simulink model "PID_DC_MOTOR_methods"  (R2016a)
settings: Solver=VariableStepAuto  StartTime=0.0  StopTime=10.0  RelTol=1e-3
InitFcn:
  | J = 0.02;
  | b = 0.05;
  | Ke = 0.1;
  | Kt = 0.2;
  | R = 3;
  | L = 0.5;
  | 
  | thetha_dot0 = 0;
  | i0 = 0;
  | 
libraries: simulink x3
settings Model: Creator=hp  LastModifiedBy=hp

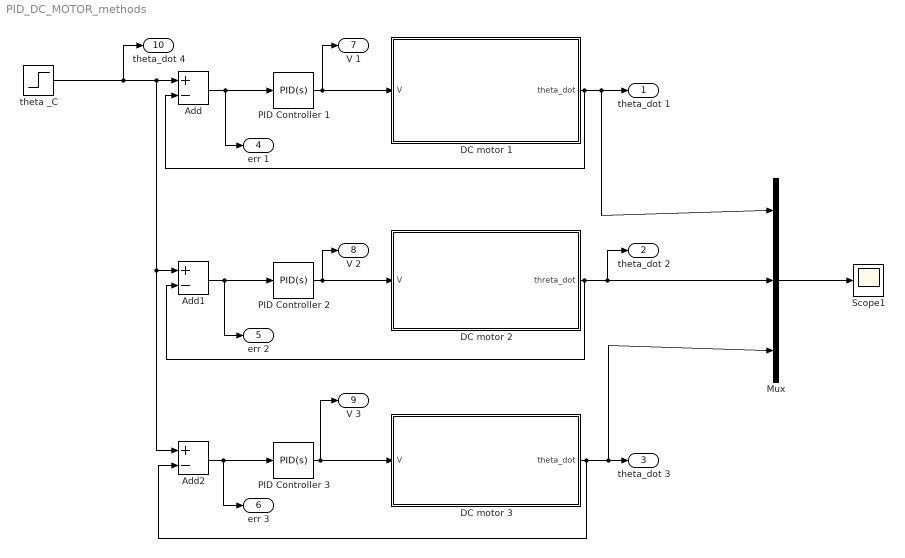
== system PID_DC_MOTOR_methods ==
  Add : Sum  Inputs=+-
  Add1 : Sum  Inputs=+-
  Add2 : Sum  Inputs=+-
  DC motor 1 : Subsystem
  DC motor 2 : Subsystem
  "DC motor 3 " : Subsystem
  Mux : Mux  Inputs=3
  PID Controller 1 : simulink/Continuous/PID Controller  Controller=PID  TimeDomain=Continuous-time  SampleTime=-1  IntegratorMethod=Forward Euler  FilterMethod=Forward Euler  Form=Parallel  UseFilter=on  ControllerParametersSource=internal  P=1.58461932315823  I=3.79137917089873  D=0.154298043345485  N=439.358617384515  InitialConditionSource=internal  InitialConditionForIntegrator=0  InitialConditionForFilter=0  ExternalReset=none  LimitOutput=off  UpperSaturationLimit=inf  LowerSaturationLimit=-inf  LinearizeAsGain=on  AntiWindupMode=none  Kb=1  TrackingMode=off  Kt=1  PParamMin=[]  PParamMax=[]  IParamMin=[]  IParamMax=[]  DParamMin=[]  DParamMax=[]  NParamMin=[]  NParamMax=[]  KbParamMin=[]  KbParamMax=[]  KtParamMin=[]  KtParamMax=[]  POutMin=[]  POutMax=[]  IOutMin=[]  IOutMax=[]  DOutMin=[]  DOutMax=[]  NOutMin=[]  NOutMax=[]  KbOutMin=[]  KbOutMax=[]  KtOutMin=[]  KtOutMax=[]  IntegratorOutMin=[]  IntegratorOutMax=[]  FilterOutMin=[]  FilterOutMax=[]  SumOutMin=[]  SumOutMax=[]  SumI1OutMin=[]  SumI1OutMax=[]  SumI2OutMin=[]  SumI2OutMax=[]  SumI3OutMin=[]  SumI3OutMax=[]  SumDOutMin=[]  SumDOutMax=[]  SaturationOutMin=[]  SaturationOutMax=[]  IntegratorContinuousStateAttributes=''  IntegratorStateMustResolveToSignalObject=off  IntegratorRTWStateStorageClass=Auto  FilterContinuousStateAttributes=''  FilterStateMustResolveToSignalObject=off  FilterRTWStateStorageClass=Auto  DifferentiatorICPrevScaledInput=0  DifferentiatorOutMin=[]  DifferentiatorOutMax=[]
  PID Controller 2 : simulink/Continuous/PID Controller  Controller=PID  TimeDomain=Continuous-time  SampleTime=-1  IntegratorMethod=Forward Euler  FilterMethod=Forward Euler  Form=Parallel  UseFilter=on  ControllerParametersSource=internal  P=1.58461932315823  I=3.79137917089873  D=0.154298043345485  N=439.358617384515  InitialConditionSource=internal  InitialConditionForIntegrator=0  InitialConditionForFilter=0  ExternalReset=none  LimitOutput=off  UpperSaturationLimit=inf  LowerSaturationLimit=-inf  LinearizeAsGain=on  AntiWindupMode=none  Kb=1  TrackingMode=off  Kt=1  PParamMin=[]  PParamMax=[]  IParamMin=[]  IParamMax=[]  DParamMin=[]  DParamMax=[]  NParamMin=[]  NParamMax=[]  KbParamMin=[]  KbParamMax=[]  KtParamMin=[]  KtParamMax=[]  POutMin=[]  POutMax=[]  IOutMin=[]  IOutMax=[]  DOutMin=[]  DOutMax=[]  NOutMin=[]  NOutMax=[]  KbOutMin=[]  KbOutMax=[]  KtOutMin=[]  KtOutMax=[]  IntegratorOutMin=[]  IntegratorOutMax=[]  FilterOutMin=[]  FilterOutMax=[]  SumOutMin=[]  SumOutMax=[]  SumI1OutMin=[]  SumI1OutMax=[]  SumI2OutMin=[]  SumI2OutMax=[]  SumI3OutMin=[]  SumI3OutMax=[]  SumDOutMin=[]  SumDOutMax=[]  SaturationOutMin=[]  SaturationOutMax=[]  IntegratorContinuousStateAttributes=''  IntegratorStateMustResolveToSignalObject=off  IntegratorRTWStateStorageClass=Auto  FilterContinuousStateAttributes=''  FilterStateMustResolveToSignalObject=off  FilterRTWStateStorageClass=Auto  DifferentiatorICPrevScaledInput=0  DifferentiatorOutMin=[]  DifferentiatorOutMax=[]
  PID Controller 3 : simulink/Continuous/PID Controller  Controller=PID  TimeDomain=Continuous-time  SampleTime=-1  IntegratorMethod=Forward Euler  FilterMethod=Forward Euler  Form=Parallel  UseFilter=on  ControllerParametersSource=internal  P=1.58461932315823  I=3.79137917089873  D=0.154298043345485  N=439.358617384515  InitialConditionSource=internal  InitialConditionForIntegrator=0  InitialConditionForFilter=0  ExternalReset=none  LimitOutput=off  UpperSaturationLimit=inf  LowerSaturationLimit=-inf  LinearizeAsGain=on  AntiWindupMode=none  Kb=1  TrackingMode=off  Kt=1  PParamMin=[]  PParamMax=[]  IParamMin=[]  IParamMax=[]  DParamMin=[]  DParamMax=[]  NParamMin=[]  NParamMax=[]  KbParamMin=[]  KbParamMax=[]  KtParamMin=[]  KtParamMax=[]  POutMin=[]  POutMax=[]  IOutMin=[]  IOutMax=[]  DOutMin=[]  DOutMax=[]  NOutMin=[]  NOutMax=[]  KbOutMin=[]  KbOutMax=[]  KtOutMin=[]  KtOutMax=[]  IntegratorOutMin=[]  IntegratorOutMax=[]  FilterOutMin=[]  FilterOutMax=[]  SumOutMin=[]  SumOutMax=[]  SumI1OutMin=[]  SumI1OutMax=[]  SumI2OutMin=[]  SumI2OutMax=[]  SumI3OutMin=[]  SumI3OutMax=[]  SumDOutMin=[]  SumDOutMax=[]  SaturationOutMin=[]  SaturationOutMax=[]  IntegratorContinuousStateAttributes=''  IntegratorStateMustResolveToSignalObject=off  IntegratorRTWStateStorageClass=Auto  FilterContinuousStateAttributes=''  FilterStateMustResolveToSignalObject=off  FilterRTWStateStorageClass=Auto  DifferentiatorICPrevScaledInput=0  DifferentiatorOutMin=[]  DifferentiatorOutMax=[]
  Scope1 : Scope
  theta _C : Step  Time=0  After=0.25  SampleTime=0
  theta_dot 1 : Outport
  theta_dot 2 : Outport  Port=2
  theta_dot 3 : Outport  Port=3
  err 1 : Outport  Port=4
  err 2 : Outport  Port=5
  err 3 : Outport  Port=6
  V 1 : Outport  Port=7
  V 2 : Outport  Port=8
  V 3 : Outport  Port=9
  theta_dot 4 : Outport  Port=10
  wires:
  DC motor 1/1(theta_dot) -> Add/2, Mux/1, theta_dot 1/1
  PID Controller 1/1 -> DC motor 1/1(V), V 1/1
  Add/1 -> err 1/1, PID Controller 1/1
  theta _C/1 -> theta_dot 4/1, Add2/1, Add1/1, Add/1
  PID Controller 2/1 -> V 2/1, DC motor 2/1(V)
  Add1/1 -> PID Controller 2/1, err 2/1
  DC motor 2/1(threta_dot) -> Add1/2, theta_dot 2/1, Mux/2
  PID Controller 3/1 -> "DC motor 3 "/1(V), V 3/1
  Add2/1 -> PID Controller 3/1, err 3/1
  "DC motor 3 "/1(theta_dot) -> Add2/2, Mux/3, theta_dot 3/1
  Mux/1 -> Scope1/1

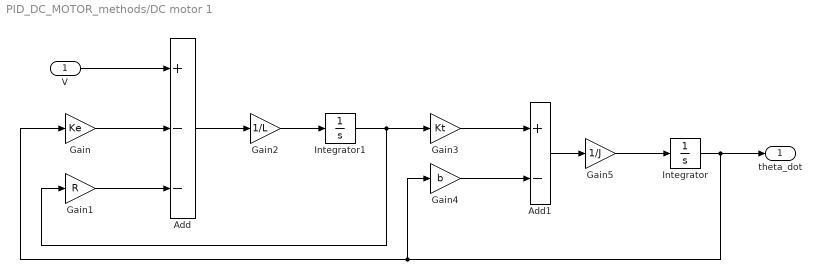
== system PID_DC_MOTOR_methods/DC motor 1 ==
  V : Inport
  Add : Sum  Inputs=+--
  Add1 : Sum  Inputs=+-
  Gain : Gain  Gain=Ke
  Gain1 : Gain  Gain=R
  Gain2 : Gain  Gain=1/L
  Gain3 : Gain  Gain=Kt
  Gain4 : Gain  Gain=b
  Gain5 : Gain  Gain=1/J
  Integrator : Integrator  InitialCondition=thetha_dot0
  Integrator1 : Integrator  InitialCondition=i0
  theta_dot : Outport
  wires:
  Integrator/1 -> theta_dot/1, Gain4/1, Gain/1
  V/1 -> Add/1
  Gain5/1 -> Integrator/1
  Gain3/1 -> Add1/1
  Gain2/1 -> Integrator1/1
  Gain1/1 -> Add/3
  Add/1 -> Gain2/1
  Add1/1 -> Gain5/1
  Gain4/1 -> Add1/2
  Integrator1/1 -> Gain1/1, Gain3/1
  Gain/1 -> Add/2

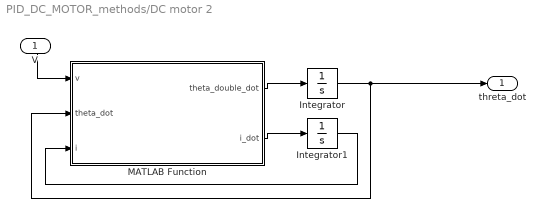
== system PID_DC_MOTOR_methods/DC motor 2 ==
  V : Inport
  Integrator : Integrator
  Integrator1 : Integrator
  MATLAB Function : MATLAB Function  TreatAsAtomicUnit=on
  threta_dot : Outport
  wires:
  MATLAB Function/1(theta_double_dot) -> Integrator/1
  MATLAB Function/2(i_dot) -> Integrator1/1
  Integrator/1 -> threta_dot/1, MATLAB Function/2(theta_dot)
  Integrator1/1 -> MATLAB Function/3(i)
  V/1 -> MATLAB Function/1(v)

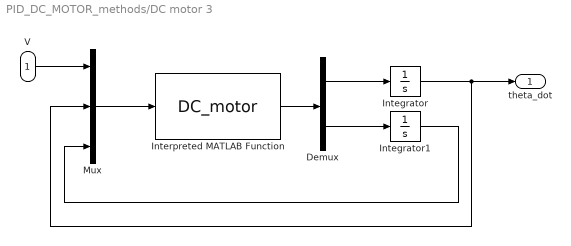
== system PID_DC_MOTOR_methods/DC motor 3  ==
  V : Inport
  Demux : Demux  Outputs=2
  Integrator : Integrator
  Integrator1 : Integrator
  Interpreted MATLAB Function : MATLABFcn  MATLABFcn=DC_motor
  Mux : Mux  Inputs=3
  theta_dot : Outport
  wires:
  Interpreted MATLAB Function/1 -> Demux/1
  Demux/1 -> Integrator/1
  Integrator/1 -> Mux/2, theta_dot/1
  V/1 -> Mux/1
  Integrator1/1 -> Mux/3
  Demux/2 -> Integrator1/1
  Mux/1 -> Interpreted MATLAB Function/1

== matlab function PID_DC_MOTOR_methods/DC motor 2/MATLAB Function ==
  data: v input; theta_double_dot output; theta_dot input; i input; i_dot output
function [theta_double_dot,i_dot] = fcn(v,theta_dot,i)
%#codegen
J = 0.02; % 
b = 0.05;
Ke = 0.1; 
Kt = 0.2;
R = 3;
L = 0.5;
theta_double_dot = (Kt *i - b * theta_dot)/J;
i_dot = (v - Ke * theta_dot - R * i) / L;
